simulink model "actuator_model"  (R2025b)
settings: Solver=VariableStepAuto  StartTime=0.0  StopTime=10.0  RelTol=1e-3
undefined symbols (not defined in the file or in its folder): pie
settings Model: Creator=issam  LastModifiedBy=issam

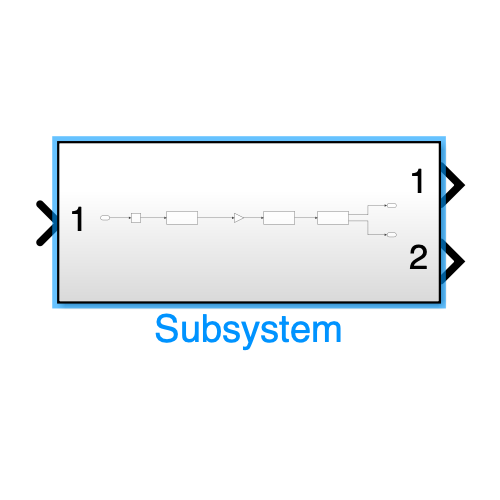
[thumbnail: Simulink's stored preview of the top-level diagram]
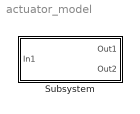
== system actuator_model ==
  Subsystem : Subsystem

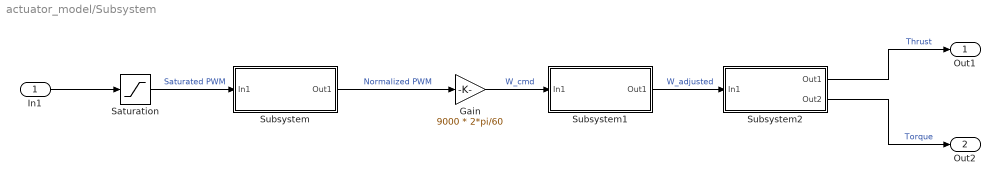
== system actuator_model/Subsystem ==
  In1 : Inport
      settings: AttributesFormatString=PWM Signal
  Gain : Gain  Gain=9000 * 2*pi/60
  Saturation : Saturate  UpperLimit=2000  LowerLimit=1000
  Subsystem : Subsystem
      settings: AttributesFormatString=Normalized PWM
  Subsystem1 : Subsystem
      settings: AttributesFormatString=Motor_dynamics
  Subsystem2 : Subsystem
      settings: AttributesFormatString=Propeller_Aerodynamics
  Out1 : Outport
      settings: AttributesFormatString=Thrust Output
  Out2 : Outport  Port=2
      settings: AttributesFormatString=Torque Output
  wires:
  In1/1 -> Saturation/1
  Saturation/1 -> Subsystem/1(In1)  "Saturated PWM"
  Subsystem/1(Out1) -> Gain/1  "Normalized PWM"
  Gain/1 -> Subsystem1/1(In1)  "W_cmd"
  Subsystem2/1(Out1) -> Out1/1  "Thrust"
  Subsystem1/1(Out1) -> Subsystem2/1(In1)  "W_adjusted"
  Subsystem2/2(Out2) -> Out2/1  "Torque"

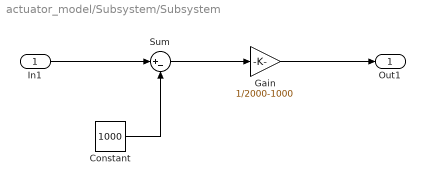
== system actuator_model/Subsystem/Subsystem ==
  In1 : Inport
      settings: AttributesFormatString=Saturated PWM
  Constant : Constant  Value=1000
  Gain : Gain  Gain=1/2000-1000
  Sum : Sum  Inputs=|+-
  Out1 : Outport
      settings: AttributesFormatString=Normalized PWM
  wires:
  In1/1 -> Sum/1
  Constant/1 -> Sum/2
  Sum/1 -> Gain/1
  Gain/1 -> Out1/1

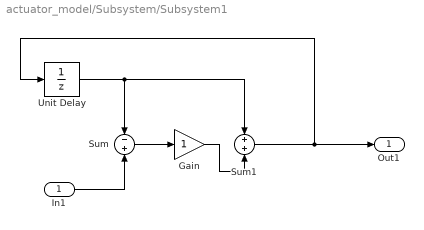
== system actuator_model/Subsystem/Subsystem1 ==
  In1 : Inport
      settings: AttributesFormatString=W_cmd
  Gain : Gain
  Sum : Sum  Inputs=-+
  Sum1 : Sum
  Unit Delay : UnitDelay  SampleTime=-1  HasFrameUpgradeWarning=on
  Out1 : Outport
      settings: AttributesFormatString=W_adjusted
  wires:
  In1/1 -> Sum/2
  Unit Delay/1 -> Sum1/1, Sum/1
  Sum/1 -> Gain/1
  Sum1/1 -> Unit Delay/1, Out1/1
  Gain/1 -> Sum1/2

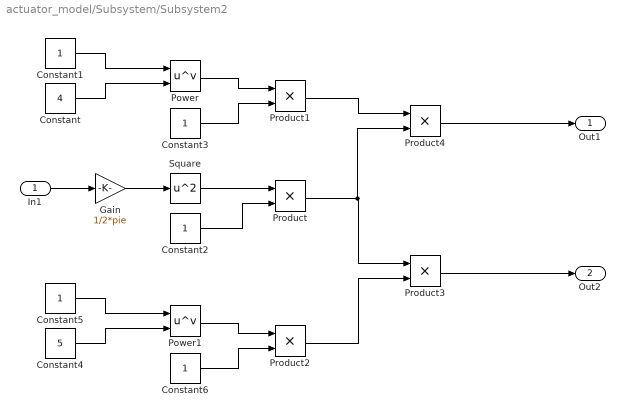
== system actuator_model/Subsystem/Subsystem2 ==
  In1 : Inport
      settings: AttributesFormatString=W_adjusted
  Constant : Constant  Value=4
  Constant{1..3,5..6} (5 alike) : Constant
      Constant1 settings: AttributesFormatString=prop_diameter
      Constant2 settings: AttributesFormatString=density
      Constant3 settings: AttributesFormatString=prop_Thrust_ratio
      Constant5 settings: AttributesFormatString=prop_diameter
      Constant6 settings: AttributesFormatString=prop_Torque_ratio
  Constant4 : Constant  Value=5
  Gain : Gain  Gain=1/2*pie
  Power : Math  Operator=pow
  Power1 : Math  Operator=pow
  Product{,1..4} (5 alike) : Product
  Square : Math  Operator=square
  Out1 : Outport
      settings: AttributesFormatString=Thrust_generated
  Out2 : Outport  Port=2
      settings: AttributesFormatString=Torque_generated
  wires:
  In1/1 -> Gain/1
  Gain/1 -> Square/1
  Constant/1 -> Power/2
  Constant1/1 -> Power/1
  Square/1 -> Product/1
  Constant2/1 -> Product/2
  Power/1 -> Product1/1
  Constant3/1 -> Product1/2
  Constant4/1 -> Power1/2
  Constant5/1 -> Power1/1
  Constant6/1 -> Product2/2
  Power1/1 -> Product2/1
  Product3/1 -> Out2/1
  Product2/1 -> Product3/2
  Product/1 -> Product4/2, Product3/1
  Product1/1 -> Product4/1
  Product4/1 -> Out1/1
